simulink subsystem "dq0_transform"  (R2024b)
settings: Solver=VariableStepAuto  StartTime=0.0  StopTime=10.0  RelTol=1e-3
settings Model: Creator=antoinedaniel  LastModifiedBy=antoinedaniel

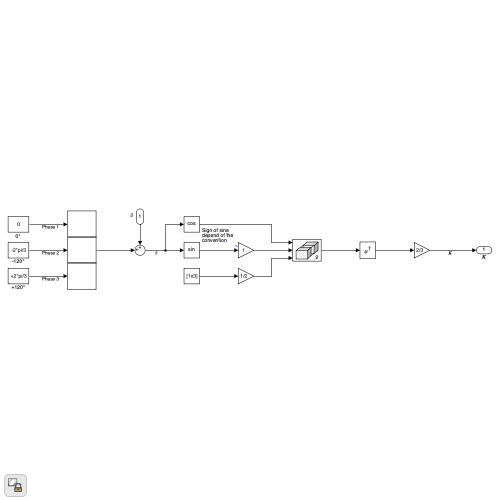
[thumbnail: Simulink's stored preview of the top-level diagram]
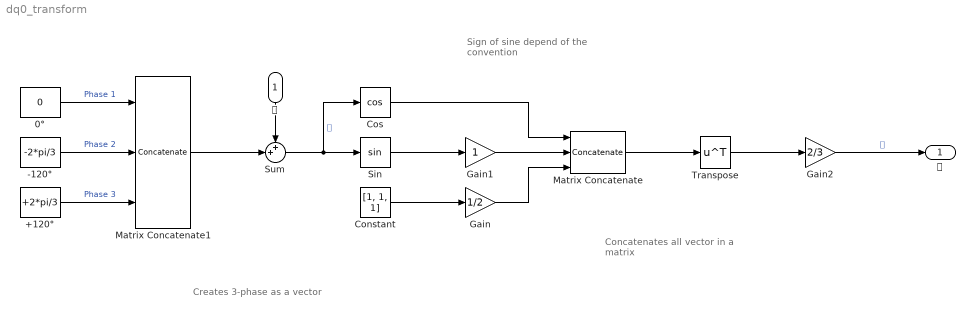
== system dq0_transform ==
  note: Sign of sine depend of the convention
  note: Creates 3-phase as a vector
  note: Concatenates all vector in a matrix
  𝜃 : Inport
  +120° : Constant  Value=+2*pi/3
  -120° : Constant  Value=-2*pi/3
  0° : Constant  Value=0
  Constant : Constant  Value=[1, 1, 1]
  Cos : Trigonometry  Operator=cos
  Gain : Gain  Gain=1/2
  Gain1 : Gain
  Gain2 : Gain  Gain=2/3
  Matrix Concatenate : Concatenate  NumInputs=3  Mode=Multidimensional array  ConcatenateDimension=2
  Matrix Concatenate1 : Concatenate  NumInputs=3  ConcatenateDimension=2
  Sin : Trigonometry
  Sum : Sum  Inputs=++|
  Transpose : Math  Operator=transpose
  𝑲 : Outport
  wires:
  Sin/1 -> Gain1/1
  +120°/1 -> Matrix Concatenate1/3  "Phase 3"
  Cos/1 -> Matrix Concatenate/1
  𝜃/1 -> Sum/1
  Matrix Concatenate/1 -> Transpose/1
  0°/1 -> Matrix Concatenate1/1  "Phase 1"
  Transpose/1 -> Gain2/1
  Matrix Concatenate1/1 -> Sum/2
  Gain/1 -> Matrix Concatenate/3
  Gain2/1 -> 𝑲/1  "𝑲"
  -120°/1 -> Matrix Concatenate1/2  "Phase 2"
  Gain1/1 -> Matrix Concatenate/2
  Sum/1 -> Cos/1, Sin/1  "𝜃"
  Constant/1 -> Gain/1
